simulink model "app_SteeringMgr"  (R2016b)
settings: Solver=FixedStepDiscrete  StartTime=0.0  StopTime=1000  FixedStep=0.001  RelTol=1e-3  EnableMultiTasking=on
PreLoadFcn:
  | try
  |    tapas_types('load');
  | catch
  |   disp('TAPAS WARNING: Tapas Types could not be loaded ...');
  | end
  | 
  | try
  |   app_types('load');
  | catch
  |   currdir =pwd;
  |   try
  |     cd('..\app_types\');
  |     app_types('load');
  |     cd(currdir);
  |   catch
  |     try
  |        cd('..\..\app_types\');
  |        app_types('load');
  |        cd(currdir);
  |     catch
  |        cd(currdir);
  |        disp('TAPAS WARNING: Application Types could not be loaded ...');
  |     end
  |   end
  |   try
  |       clear currdir;
  |   catch
  |      %Do nothing
  |   end
  | end
settings Model: Creator=kmansour  LastModifiedBy=kmansour
settings DataIOCC: LimitDataPoints=on  SaveFormat=Array
settings OptimizationCC: LifeSpan=1
settings DebuggingCC: AllowSymbolicDim=off  SFUnexpectedBacktrackingDiag=warning  SFNoUnconditionalDefaultTransitionDiag=warning  SFExecutionAtInitializationDiag=none
settings HardwareCC: ProdBitPerPointer=32  ProdBitPerSizeT=32  ProdBitPerPtrDiffT=32  ProdLargestAtomicFloat=None  ProdIntDivRoundTo=Undefined  ProdEndianess=Unspecified  ProdWordSize=32  ProdHWDeviceType=32-bit Generic
settings ModelReferenceCC: ModelReferenceNumInstancesAllowed=Single  PropagateSignalLabelsOutOfModel=off
settings RTWCC: SystemTargetFile=ert.tlc  GenCodeOnly=on  TemplateMakefile=ert_default_tmf  Description=Embedded Coder  GenerateReport=on  CustomSourceCode="#include \"rte.h\""  IncludeHyperlinkInReport=on  LaunchReport=on  GenerateTraceInfo=on  GenerateTraceReport=on  GenerateTraceReportSl=on  GenerateTraceReportSf=on  GenerateTraceReportEml=on
settings CodeAppCC: IgnoreCustomStorageClasses=off  MaxIdLength=63
settings ERTTargetCC: GenerateSampleERTMain=on  ERTSrcFileBannerTemplate=tapas_code_template.cgt  ERTHdrFileBannerTemplate=tapas_code_template.cgt  ERTDataSrcFileTemplate=tapas_code_template.cgt  ERTDataHdrFileTemplate=tapas_code_template.cgt  ERTCustomFileTemplate=example_file_process.tlc  ConvertIfToSwitch=off  SuppressUnreachableDefaultCases=off
settings ConfigComp: CovMetricSettings=dw  CovHtmlReporting=on  CovSaveCumulativeToWorkspaceVar=on  CovSaveSingleToWorkspaceVar=on  CovExternalEMLEnable=off

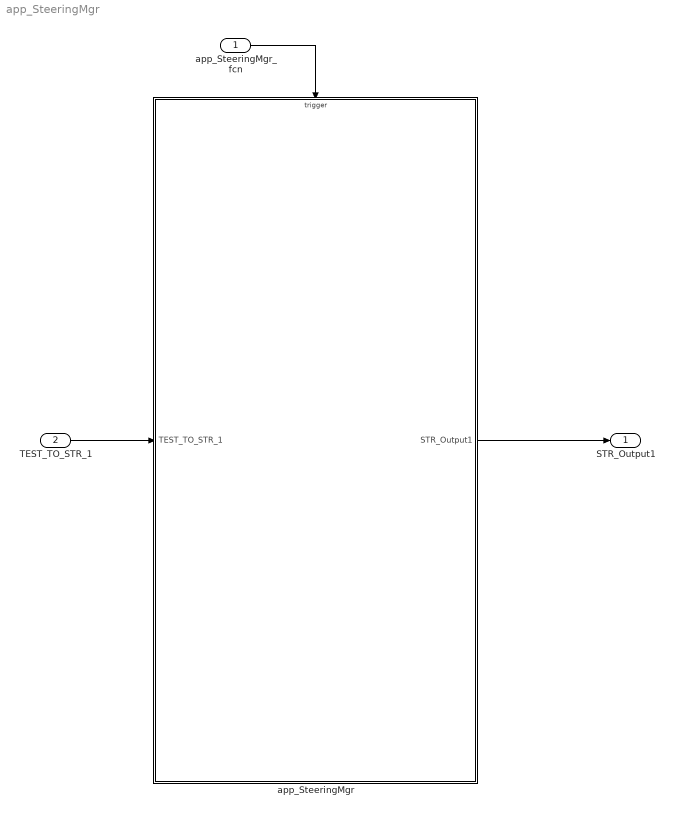
== system app_SteeringMgr ==
  app_SteeringMgr_fcn : Inport  SampleTime=10e-3  OutputFunctionCall=on
  TEST_TO_STR_1 : Inport  Port=2
  app_SteeringMgr : Subsystem
  STR_Output1 : Outport
  wires:
  app_SteeringMgr_fcn/1 -> app_SteeringMgr/Trigger
  TEST_TO_STR_1/1 -> app_SteeringMgr/1(TEST_TO_STR_1)
  app_SteeringMgr/1(STR_Output1) -> STR_Output1/1

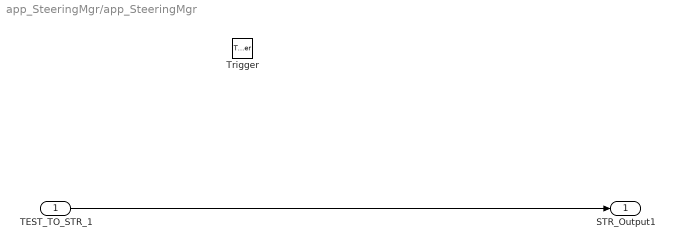
== system app_SteeringMgr/app_SteeringMgr ==
  TEST_TO_STR_1 : Inport
  Trigger : TriggerPort  TriggerType=function-call  VariantControl=Variant  SampleTimeType=periodic  SampleTime=-1  PortDimensions=1
  STR_Output1 : Outport
  wires:
  TEST_TO_STR_1/1 -> STR_Output1/1
